simulink model "SquareWaveSumOfSineWaves_MathFunction"  (R2015b)
settings: Solver=VariableStepAuto  StartTime=0.0  StopTime=100.0  MaxStep=0.001  MinStep=0.001  RelTol=1e-3
settings Model: Creator=mihai.ciobanu  LastModifiedBy=mihai.ciobanu

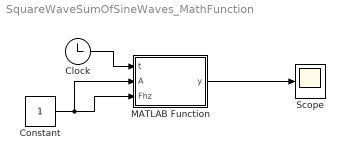
== system SquareWaveSumOfSineWaves_MathFunction ==
  Clock : Clock
  Constant : Constant
  MATLAB Function : MATLAB Function  TreatAsAtomicUnit=on
  Scope : Scope
  wires:
  Constant/1 -> MATLAB Function/2(A), MATLAB Function/3(Fhz)
  Clock/1 -> MATLAB Function/1(t)
  MATLAB Function/1(y) -> Scope/1

== matlab function SquareWaveSumOfSineWaves_MathFunction/MATLAB Function ==
  data: t input; A input; Fhz input; y output
function y = fcn(t,A,Fhz)
%#codegen
Frad = Fhz/(2*pi);
y = A*sin(Frad*t);
